simulink model "partFiveUnicycle"  (R2021b)
settings: Solver=VariableStepAuto  StartTime=0.0  StopTime=10  RelTol=1e-3
settings Model: Creator=ericp  LastModifiedBy=ericp

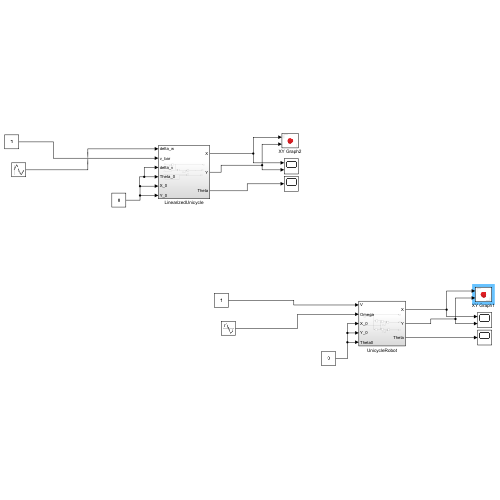
[thumbnail: Simulink's stored preview of the top-level diagram]
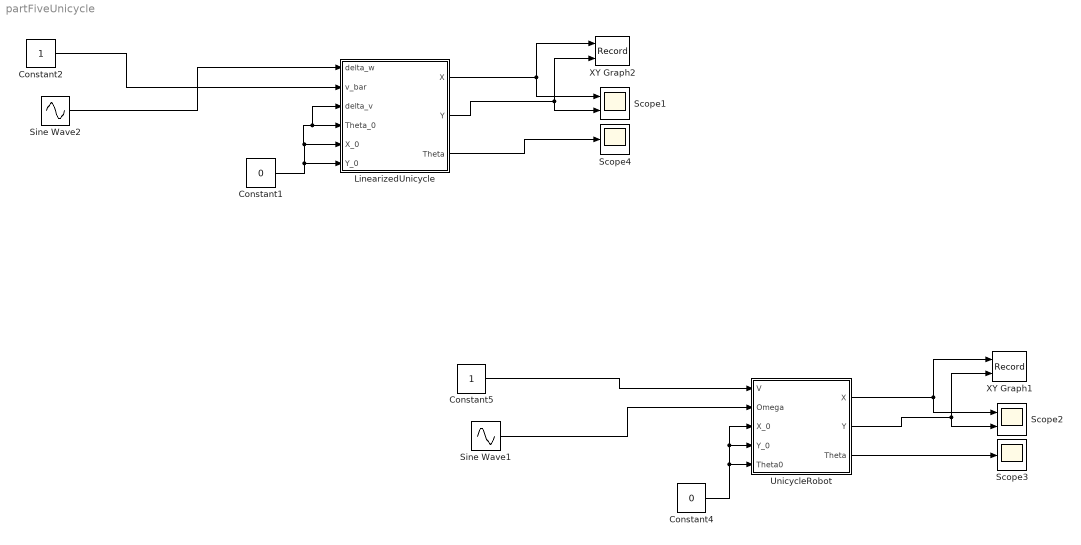
== system partFiveUnicycle ==
  Constant1 : Constant  Value=0
  Constant2 : Constant
  Constant4 : Constant  Value=0
  Constant5 : Constant
  LinearizedUnicycle : Subsystem
  Scope1 : Scope  NumInputPorts=2
  Scope2 : Scope  NumInputPorts=2
  Scope3 : Scope
  Scope4 : Scope
  Sine Wave1 : Sin  Frequency=0.01  SampleTime=0
  Sine Wave2 : Sin  Frequency=0.01  SampleTime=0
  UnicycleRobot : Subsystem
  XY Graph1 : Record  FileSettingsInternal="{\"entries\":[{\"content\":{\"excelSettings\":{\"content\":{},\"type\":\"Streamout.ExcelSettings\"}},\"type\":\"Streamout.FileSettingStorage\",\"uuid\":\"d30338bd-7ee8-4782-be17-cb4409a8a6bc\"}],\"packageUris\":[\"http://schema.mathworks.com/mf0/streamout_blocks/R2020a\"],\"version\":\"1.0\"}"  Layout=[1 1]  SignalsInternal="{\"entries\":[{\"content\":{\"signals\":[{\"content\":{\"blockPath\":[\"partFiveUnicycle/XY Graph1\"],\"channel\":[],\"dimensions\":[1],\"domain\":\"partFiveUnicycle/XY Graph1\",\"lineColor\":\"#a2142f\",\"plots\":[1],\"port\":1,\"sid\":[\"\"],\"signalID\":1457,\"signalName\":\"UnicycleRobot:1\"},\"type\":\"RecordBlkView.Signal\",\"uuid\":\"c9e693ce-a278-47cb-b660-ac0b0165f9a6\"},{\"content\":{\"blockPath\":[\"partFiveUnicycle/XY Graph1\"],\"channel\":[],\"dimensions\":[1],\"domain\":\"partFiveUnicycle/XY Graph1\",\"lineColor\":\"#139fff\",\"plots\":[1],\"port\":2,\"sid\":[\"\"],\"signalID\":1461,\"signalName\":\"UnicycleRobot:2\"},\"type\":\"RecordBlkView.Signal\",\"uuid\":\"66159780-c29d-4727-80f2-5395887d84aa\"}]},\"type\":\"RecordBlkView.InputSignals\",\"uuid\":\"d28b59ed-fb91-40ea-9f1f-cd4479eb6b41\"}],\"packageUris\":[\"http://schema.mathworks.com/mf0/streamout_blocks/R2020a\"],\"version\":\"1.0\"}"  VisualizationBindings="{\"xyplotplugin\":{\"info\":[{\"series\":[{\"bindingParametersList\":[{\"parameter\":\"X-Axis\",\"signalID\":1457,\"signalName\":\"UnicycleRobot:1\"},{\"parameter\":\"Y-Axis\",\"signalID\":1461,\"signalName\":\"UnicycleRobot:2\"}],\"seriesID\":479}],\"subplotID\":1}]}}"  CompatibilityTag=XY
  XY Graph2 : Record  FileSettingsInternal="{\"entries\":[{\"content\":{\"excelSettings\":{\"content\":{},\"type\":\"Streamout.ExcelSettings\"}},\"type\":\"Streamout.FileSettingStorage\",\"uuid\":\"c50187c0-4f9a-4e6e-aa36-18cb240b89f3\"}],\"packageUris\":[\"http://schema.mathworks.com/mf0/streamout_blocks/R2020a\"],\"version\":\"1.0\"}"  Layout=[1 1]  SignalsInternal="{\"entries\":[{\"content\":{\"signals\":[{\"content\":{\"blockPath\":[\"partFiveUnicycle/XY Graph2\"],\"channel\":[],\"dimensions\":[1],\"domain\":\"partFiveUnicycle/XY Graph2\",\"lineColor\":\"#a2142f\",\"plots\":[1],\"port\":1,\"sid\":[\"\"],\"signalID\":1449,\"signalName\":\"LinearizedUnicycle:1\"},\"type\":\"RecordBlkView.Signal\",\"uuid\":\"baf5c45d-050c-4e9d-8829-edaf485a6333\"},{\"content\":{\"blockPath\":[\"partFiveUnicycle/XY Graph2\"],\"channel\":[],\"dimensions\":[1],\"domain\":\"partFiveUnicycle/XY Graph2\",\"lineColor\":\"#139fff\",\"plots\":[1],\"port\":2,\"sid\":[\"\"],\"signalID\":1453,\"signalName\":\"LinearizedUnicycle:2\"},\"type\":\"RecordBlkView.Signal\",\"uuid\":\"91153072-bcf6-4b35-ab13-871dbe226c91\"}]},\"type\":\"RecordBlkView.InputSignals\",\"uuid\":\"c69012d5-8d48-4a44-8b04-ca73451734df\"}],\"packageUris\":[\"http://schema.mathworks.com/mf0/streamout_blocks/R2020a\"],\"version\":\"1.0\"}"  VisualizationBindings="{\"xyplotplugin\":{\"info\":[{\"series\":[{\"bindingParametersList\":[{\"parameter\":\"Y-Axis\",\"signalID\":1453,\"signalName\":\"LinearizedUnicycle:2\"},{\"parameter\":\"X-Axis\",\"signalID\":1453,\"signalName\":\"LinearizedUnicycle:2\"}],\"seriesID\":56809}],\"subplotID\":1}]}}"  CompatibilityTag=XY
  wires:
  UnicycleRobot/3(Theta) -> Scope3/1
  UnicycleRobot/1(X) -> XY Graph1/1, Scope2/1
  UnicycleRobot/2(Y) -> XY Graph1/2, Scope2/2
  Constant4/1 -> UnicycleRobot/5(Theta0), UnicycleRobot/4(Y_0), UnicycleRobot/3(X_0)
  Constant5/1 -> UnicycleRobot/1(V)
  Sine Wave1/1 -> UnicycleRobot/2(Omega)
  Constant2/1 -> LinearizedUnicycle/2(v_bar)
  Constant1/1 -> LinearizedUnicycle/5(X_0), LinearizedUnicycle/3(delta_v), LinearizedUnicycle/4(Theta_0), LinearizedUnicycle/6(Y_0)
  Sine Wave2/1 -> LinearizedUnicycle/1(delta_w)
  LinearizedUnicycle/1(X) -> Scope1/1, XY Graph2/1
  LinearizedUnicycle/3(Theta) -> Scope4/1
  LinearizedUnicycle/2(Y) -> XY Graph2/2, Scope1/2

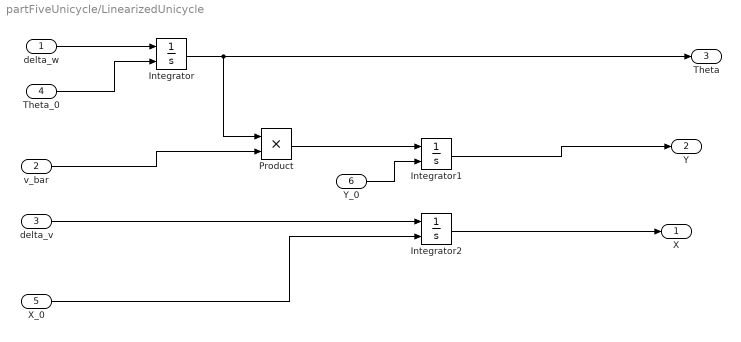
== system partFiveUnicycle/LinearizedUnicycle ==
  delta_w : Inport
  v_bar : Inport  Port=2
  delta_v : Inport  Port=3
  Theta_0 : Inport  Port=4
  X_0 : Inport  Port=5
  Y_0 : Inport  Port=6
  Integrator : Integrator  InitialConditionSource=external
  Integrator1 : Integrator  InitialConditionSource=external
  Integrator2 : Integrator  InitialConditionSource=external
  Product : Product
  X : Outport
  Y : Outport  Port=2
  Theta : Outport  Port=3
  wires:
  Integrator/1 -> Theta/1, Product/1
  Theta_0/1 -> Integrator/2
  v_bar/1 -> Product/2
  Product/1 -> Integrator1/1
  delta_w/1 -> Integrator/1
  X_0/1 -> Integrator2/2
  Integrator1/1 -> Y/1
  Y_0/1 -> Integrator1/2
  delta_v/1 -> Integrator2/1
  Integrator2/1 -> X/1

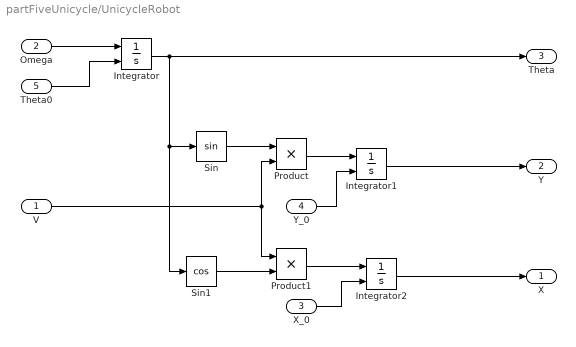
== system partFiveUnicycle/UnicycleRobot ==
  V : Inport
  Omega : Inport  Port=2
  X_0 : Inport  Port=3
  Y_0 : Inport  Port=4
  Theta0 : Inport  Port=5
  Integrator : Integrator  InitialConditionSource=external
  Integrator1 : Integrator  InitialConditionSource=external
  Integrator2 : Integrator  InitialConditionSource=external
  Product : Product
  Product1 : Product
  Sin : Trigonometry
  Sin1 : Trigonometry  Operator=cos
  X : Outport
  Y : Outport  Port=2
  Theta : Outport  Port=3
  wires:
  Sin1/1 -> Product1/2
  V/1 -> Product1/1, Product/2
  Integrator/1 -> Theta/1, Sin1/1, Sin/1
  Integrator2/1 -> X/1
  Sin/1 -> Product/1
  Theta0/1 -> Integrator/2
  Y_0/1 -> Integrator1/2
  Omega/1 -> Integrator/1
  X_0/1 -> Integrator2/2
  Integrator1/1 -> Y/1
  Product1/1 -> Integrator2/1
  Product/1 -> Integrator1/1
